simulink library "imageUDPNode_ul"  (R2018b)
settings: Solver=VariableStepAuto  StartTime=0.0  StopTime=10.0  RelTol=1e-3
undefined symbols (not defined in the file or in its folder): ipaddr, PTP, udpslgate
libraries: ptplib x5, xpcutilitieslib x1
settings Model: Creator=MAE-NCSUCORE  LastModifiedBy=MAE-NCSUCORE

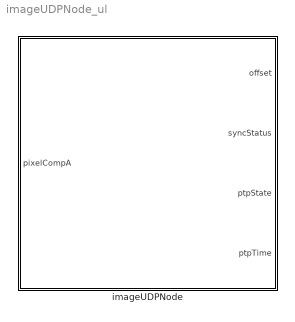
== system imageUDPNode_ul ==
  imageUDPNode : Subsystem  TreatAsAtomicUnit=on  mask{sample_time=0.025, IpAddress=30.30.30.1, toPort=8001, offset_threshold=250e-6, sync_interval=0.2, min_pdelay_req_interval=2, MaskUnpackedDataTypes={['double']}}
      mask prompts: sample_time "Sample time (-1 for inherited)"; IpAddress "IP address:"; toPort "To port:"; offset_threshold "Offset threshold (second)"; sync_interval "Sync interval (second):"; min_pdelay_req_interval "Min delay or pdelay request interval (second):"; MaskUnpackedDataTypes "Input port (unpacked) data types (cell array):"
      mask init:
      | imageUDPNode;
      mask TypeOptions sample_time: IEEE 1588 Read Offset/sample_time | IEEE 1588 Read State/sample_time | IEEE 1588 Read Time/sample_time | IEEE 1588 Real-Time UDP/sample_time | IEEE 1588 Sync Status/sample_time | UDP Send/sampleTime
      mask TypeOptions IpAddress: IEEE 1588 Real-Time UDP/IpAddress
      mask TypeOptions toPort: UDP Send/toPort
      mask TypeOptions offset_threshold: IEEE 1588 Sync Status/offset_threshold
      mask TypeOptions sync_interval: IEEE 1588 Real-Time UDP/sync_interval
      mask TypeOptions min_pdelay_req_interval: IEEE 1588 Real-Time UDP/min_pdelay_req_interval
      mask TypeOptions MaskUnpackedDataTypes: Byte Packing/MaskUnpackedDataTypes

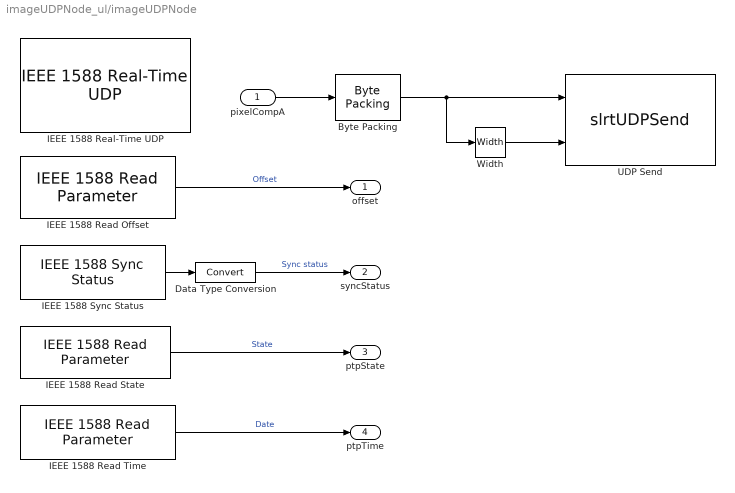
== system imageUDPNode_ul/imageUDPNode ==
  pixelCompA : Inport
  Byte Packing : xpcutilitieslib/Byte Packing   MaskPackedDataType=uint8  MaskUnpackedDataTypes=MaskUnpackedDataTypes  MaskAlignment=1
  Data Type Conversion : DataTypeConversion
  IEEE 1588 Read Offset : ptplib/IEEE 1588 Read Parameter  Priority=1  ID=1  param=Offset from Master  sample_time=sample_time  enable_read_precision=off
      settings: SourceProductName=Simulink Real-Time  SourceProductBaseCode=XP
  IEEE 1588 Read State : ptplib/IEEE 1588 Read Parameter  Priority=1  ID=1  param=Protocol state  sample_time=sample_time  enable_read_precision=off
      settings: SourceProductName=Simulink Real-Time  SourceProductBaseCode=XP
  IEEE 1588 Read Time : ptplib/IEEE 1588 Read Parameter  Priority=1  ID=1  param=PTP time (time-of-day)  sample_time=sample_time  enable_read_precision=off
      settings: SourceProductName=Simulink Real-Time  SourceProductBaseCode=XP
  IEEE 1588 Real-Time UDP : ptplib/IEEE 1588 Real-Time UDP  Priority=0  ID=1  PciBus=4  PciSlot=0  PciFunction=0  time_inc=4000000  sample_time=sample_time  IpSource=Specify  IpAddress=30.30.30.1  SubnetMask=255.255.255.0  Gateway=0.0.0.0  Receive1=30.30.30.30  dest_ip_select=Standard PTP multicast (224.0.1.129, 224.0.0.107)  custom_dest_ip_addr=30.30.30.30  MulticastList=[ipaddr('224.0.1.129'), ipaddr('224.0.0.107')]  Multicast={macaddr('01:00:5E:00:01:81'), macaddr('01:00:5E:00:00:6B')}  time_source=Ethernet board  timescale=PTP (1970-01-01)  epoch=[1970 01 01 00]  delay_measure=Request-response  slave_only=off  enable_advanced_config=on  domain_num=0  utc_offset=35  priority1=128  clock_class=248  clock_accuracy=hex2dec('FE')  priority2=128  announce_interval=2  sync_interval=sync_interval  min_pdelay_req_interval=min_pdelay_req_interval  announce_receipt_timeout=30
      settings: SourceProductName=Simulink Real-Time  SourceProductBaseCode=XP
  IEEE 1588 Sync Status : ptplib/IEEE 1588 Sync Status  Priority=1  ID=1  offset_threshold=offset_threshold  sample_time=sample_time
      settings: SourceProductName=Simulink Real-Time  SourceProductBaseCode=XP
  UDP Send : S-Function  AncestorBlock=xpcrtudplib/UDP Send  LoadFcn=udpslgate('privateupdateIPlist', gcb, 'SetIPAddress');  InitFcn=|  FunctionName=slrtUDPSend  Parameters=ipAddress, localPort, toAdd, toPort, useHostTargetComm, sampleTime  SFunctionDeploymentMode=off  EnableBusSupport=off  mask(slrtudpsend){ipAddress=Use host-target connection, ipAddressVal=Use host-target connection, localPort=-1, toAddress=30.30.30.30, toPort=toPort, sampleTime=sample_time}
      | % Validate model
      | udpvalidatemodel(gcb);
      | ipAddress_init(gcb,gcs);
      mask prompts: ipAddress "Local IP address:"; ipAddressVal "Local IP address:"; localPort "Local port:"; toAddress "To IP address:"; toPort "To port:"; sampleTime "Sample time (-1 for inherited):"
      mask help:
      | Send data over UDP network to a remote device. Send to 255.255.255.255 for broadcast.
      |
      | 'Local IP address' applies only when the block executes on a target computer.
      mask init:
      | % Update ipAddress popup options
      | udpslgate('privateupdateIPlist', gcb, 'UpdateIPList');
      | 
      | % Validate mask parameter values
      | [toAdd, useHostTargetComm] = ...
      |     udpslgate('privateUDPSend', 'validateParams', ipAddress, localPort, toAddress, toPort);
      settings: PreSaveFcn=udpslgate('privateupdateIPlist', gcb, 'UpdateIpAddressVal');
      mask Help: eval('xpcdoc(''UDP_Send'')');
      mask TypeOptions ipAddress: Use host-target connection | 30.30.30.1
      mask Callback ipAddress: udpslgate('privateupdateIPlist', gcb, 'UpdateIPList');
      mask DialogControl DescGroupVar Prompt: UDP Send
      mask Display:
      | maskDisplay = udpslgate('privateUDPSend', 'dispStr', ipAddress, localPort, toAddress, toPort);
      | disp(maskDisplay)
      | 
      | port_label('input', 1, 'Data')
      | port_label('input', 2, 'Length')
  Width : Width
  offset : Outport
  syncStatus : Outport  Port=2
  ptpState : Outport  Port=3
  ptpTime : Outport  Port=4
  wires:
  IEEE 1588 Read Offset/1 -> offset/1  "Offset"
  IEEE 1588 Read State/1 -> ptpState/1  "State"
  Byte Packing/1 -> Width/1, UDP Send/1
  IEEE 1588 Sync Status/1 -> Data Type Conversion/1
  IEEE 1588 Read Time/1 -> ptpTime/1  "Date"
  Data Type Conversion/1 -> syncStatus/1  "Sync status"
  Width/1 -> UDP Send/2
  pixelCompA/1 -> Byte Packing/1
